simulink model "IMcontrol0"  (Simulink 10.1)
settings: Solver=ode23tb  StartTime=0.0  StopTime=10  MaxStep=1e-4  RelTol=1e-3
undefined symbols (not defined in the file or in its folder): DiscIntNeverNeededParam, Ts
libraries: powerlib x4, simulink x1
settings Model: Creator=80573  LastModifiedBy=Lenovo
settings DataIOCC: SaveFormat=Dataset
settings OptimizationCC: LifeSpan=auto
settings DebuggingCC: UnderspecifiedInitializationDetection=Simplified  MergeDetectMultiDrivingBlocksExec=error  SFUnexpectedBacktrackingDiag=error  SFNoUnconditionalDefaultTransitionDiag=error  SFExecutionAtInitializationDiag=warning
settings HardwareCC: ProdBitPerPointer=64  ProdBitPerSizeT=64  ProdBitPerPtrDiffT=64  ProdLargestAtomicFloat=Float  ProdIntDivRoundTo=Zero  ProdEndianess=LittleEndian  ProdWordSize=64  ProdHWDeviceType=Intel->x86-64 (Windows64)
settings ModelReferenceCC: PropagateSignalLabelsOutOfModel=on
settings CodeAppCC: StateflowObjectComments=off
settings GRTTargetCC: TargetLangStandard=C99 (ISO)  CombineOutputUpdateFcns=on  GRTInterface=off
settings ConfigComp: CovMetricSettings=dwe  CovHtmlReporting=off  CovSaveCumulativeToWorkspaceVar=off  CovSaveSingleToWorkspaceVar=off  CovExternalEMLEnable=on

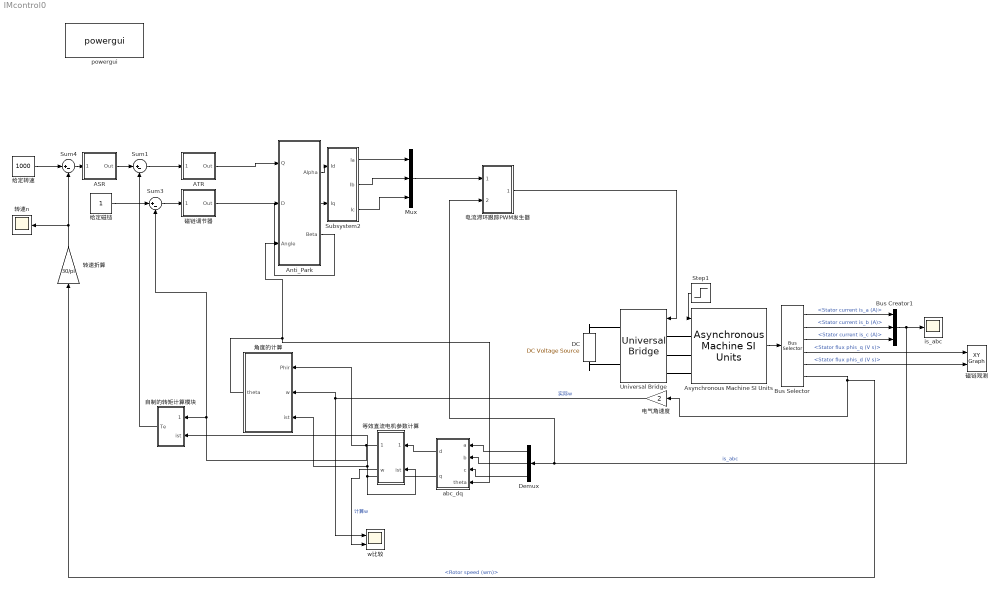
== system IMcontrol0 ==
  ASR : Subsystem  AncestorBlock=|  DialogController=POWERSYS.PowerSysDialog  mask(Discrete PI Controller){Kpw=3.8, Kiw=0.8, Ba=0, Par_Limits=[30 -30], Init=0, Ts=Ts}
      | powerlib_extras/Discrete 
      | Control Blocks/Discrete
      | PI Controller
      mask prompts: Kpw "Proportional gain (Kp):"; Kiw "Integral gain (Ki):"; Ba "feedback gain (Ba)"; Par_Limits "Output limits: [ Upper   Lower ]"; Init "Output initial value:"; Ts "Sample time:"
      mask help: This block implements a discrete PI controller.
      mask init:
      | UpperLimit=Par_Limits(1);
      | LowerLimit=Par_Limits(2);
      | power_initmask();
      mask Help: This block is part of a subset of blocks in the Extras library that does not have documentation associated with it, other than the block mask description.
      mask Display: disp('PI');
  ATR : Subsystem  AncestorBlock=|  DialogController=POWERSYS.PowerSysDialog  mask(Discrete PI Controller){Kpw=4.5, Kiw=12, Ba=0, Par_Limits=[60 -60], Init=0, Ts=Ts}
      | powerlib_extras/Discrete 
      | Control Blocks/Discrete
      | PI Controller
      mask prompts: Kpw "Proportional gain (Kp):"; Kiw "Integral gain (Ki):"; Ba "feedback gain (Ba)"; Par_Limits "Output limits: [ Upper   Lower ]"; Init "Output initial value:"; Ts "Sample time:"
      mask help: This block implements a discrete PI controller.
      mask init:
      | UpperLimit=Par_Limits(1);
      | LowerLimit=Par_Limits(2);
      | power_initmask();
      mask Help: This block is part of a subset of blocks in the Extras library that does not have documentation associated with it, other than the block mask description.
      mask Display: disp('PI');
  Anti_Park : Subsystem
  Asynchronous Machine SI Units : powerlib/Machines/Asynchronous Machine SI Units  RotorType=Squirrel-cage  PresetModel=No  MechanicalLoad=Torque Tm  ShowDetailedParameters=on  ReferenceFrame=Stationary  Units=SI  MeasurementBus=off  NominalParameters=[7500 380 50]  Stator=[0.7384 0.003045]  Rotor=[0.07402 0.003045]  Cage1=[0.4155 0.002066]  Cage2=[0.4168 0.0003495]  Lm=0.1241  Mechanical=[0.0343 0 2]  PolePairs=2  InitialConditions=[1 0 0 0 0 0 0 0]  SimulateSaturation=off  Saturation=[14.03593122, 27.81365428, 53.79336849, 72.68890987, 97.98006896, 148.6815601, 215.7428561, 302.9841135, 428.7778367 ; 230, 322, 414, 460, 506, 552, 598, 644, 690]  LoadFlowParameters=1492000  TsPowergui=0  TsBlock=-1  IterativeModel=Trapezoidal non iterative  IterativeDiscreteModel=Trapezoidal non iterative  Pmec=1.492e+006
  Bus Creator1 : BusCreator  Inputs=3
  Bus Selector : BusSelector  OutputSignals=Stator measurements.Stator current is_a (A),Stator measurements.Stator current is_b (A),Stator measurements.Stator current is_c (A),Stator measurements.Stator flux phis_q (V s),Stator measurements.Stator flux phis_d (V s),Mechanical.Rotor speed (wm)
  DC : powerlib/Electrical Sources/DC Voltage Source  Amplitude=510  Measurements=None
  Demux : Demux  Outputs=3
  Mux : Mux  Inputs=3
  Step1 : Step  After=2  SampleTime=0
  Subsystem2 : Subsystem
  Sum1 : Sum  Inputs=|+-
  Sum3 : Sum  Inputs=|+-
  Sum4 : Sum  Inputs=|+-
  Universal Bridge : powerlib/Power Electronics/Universal Bridge  Arms=3  SnubberResistance=1e5  SnubberCapacitance=inf  Device=IGBT / Diodes  Ron=1e-3  Lon=0  ForwardVoltages="[  0  0  ]"  ForwardVoltage=0  GTOparameters=[ 10e-6 , 20e-6 ]  IGBTparameters=[ 1e-6 , 2e-6 ]  Measurements=None  Measurements_2=None  converterType=Rectifier
  abc_dq : Subsystem
  is_abc : Scope
  powergui : powerlib/powergui  SimulationMode=Discrete  SampleTime=0.00001  frequency=50  Iterations=50  frequencyindice=50  Pbase=100e6  ErrMax=1e-4  UnitsV=kV  UnitsW=MW  buscounter=0  FunctionMessages=off  echomessages=off  EnableUseOfTLC=off  CurrentSourceSwitches=off  DisableSnubberDevices=off  DisableRonSwitches=off  DisableVfSwitches=off  DisplayEquations=off  AutomaticDiscreteSolvers=off  SolverType=Tustin/Backward Euler (TBE)  Interpol=off  ExternalGateDelay=off  methode=off  Ts=100  x0status=zero  SPID=on  SwTol=0  HookPort=off  NonlinearTolerance=1e-4  nMaxIteration=100  ContinueOnMaxIteration=off  RestoreLinks=warning  ResistiveCurrentMeasurement=off  Frange=[0:2:500]  Ylog=off  Xlog=on  ShowGrid=off  save=off  variable=ZData  structure=0  ZoomFFT=on  StartTime=0.0  cycles=1  DisplayStyle=1  fundamental=60  FreqAxis=off  MaxFrequency=1000  frequencyindicesteady=1  RmsSteady=1  display=off
  w比较 : Scope  NumInputPorts=2
  电气角速度 : Gain  Gain=2
  电流滞环跟踪PWM发生器 : Subsystem
  磁链观测 : simulink/Sinks/XY Graph  xmin=-1  xmax=1  ymin=-1  ymax=1  st=-1
  磁链调节器 : Subsystem  AncestorBlock=|  DialogController=POWERSYS.PowerSysDialog  mask(Discrete PI Controller){Kpw=1.8, Kiw=100, Ba=0, Par_Limits=[13 -13], Init=0, Ts=Ts}
      | powerlib_extras/Discrete 
      | Control Blocks/Discrete
      | PI Controller
      mask prompts: Kpw "Proportional gain (Kp):"; Kiw "Integral gain (Ki):"; Ba "feedback gain (Ba)"; Par_Limits "Output limits: [ Upper   Lower ]"; Init "Output initial value:"; Ts "Sample time:"
      mask help: This block implements a discrete PI controller.
      mask init:
      | UpperLimit=Par_Limits(1);
      | LowerLimit=Par_Limits(2);
      | power_initmask();
      mask Help: This block is part of a subset of blocks in the Extras library that does not have documentation associated with it, other than the block mask description.
      mask Display: disp('PI');
  等效直流电机参数计算 : Subsystem
  给定磁链 : Constant
  给定转速 : Constant  Value=1000
  自制的转矩计算模块 : Subsystem
  角度的计算 : Subsystem
  转速n : Scope
  转速折算 : Gain  Gain=30/pi
  wires:
  Step1/1 -> Asynchronous Machine SI Units/1
  abc_dq/1(d) -> 等效直流电机参数计算/1(ism)
  abc_dq/2(q) -> 自制的转矩计算模块/2(ist), 角度的计算/3(ist), 等效直流电机参数计算/2(ist)
  Sum1/1 -> ATR/1(Error)
  Sum3/1 -> 磁链调节器/1(Error)
  Sum4/1 -> ASR/1(Error)
  给定磁链/1 -> Sum3/1
  等效直流电机参数计算/1(Phir) -> 角度的计算/1(Phir), 自制的转矩计算模块/1(phir), Sum3/2
  Mux/1 -> 电流滞环跟踪PWM发生器/1(Iabc*)
  角度的计算/1(theta) -> Anti_Park/3(Angle), abc_dq/4(theta)
  Subsystem2/1(Ia) -> Mux/1
  Bus Selector/1 -> Bus Creator1/1  "<Stator current is_a (A)>"
  Bus Selector/3 -> Bus Creator1/3  "<Stator current is_c (A)>"
  Bus Selector/4 -> 磁链观测/1  "<Stator flux phis_q (V s)>"
  Bus Selector/5 -> 磁链观测/2  "<Stator flux phis_d (V s)>"
  Bus Selector/2 -> Bus Creator1/2  "<Stator current is_b (A)>"
  Bus Selector/6 -> 转速折算/1, 电气角速度/1  "<Rotor speed (wm)>"
  Bus Creator1/1 -> 电流滞环跟踪PWM发生器/2(Iabc), Demux/1, is_abc/1  "is_abc"
  Asynchronous Machine SI Units/1 -> Bus Selector/1
  电流滞环跟踪PWM发生器/1(pulse) -> Universal Bridge/1
  Demux/2 -> abc_dq/2(b)
  Demux/3 -> abc_dq/3(c)
  Demux/1 -> abc_dq/1(a)
  电气角速度/1 -> w比较/1, 角度的计算/2(w)  "实际w"
  等效直流电机参数计算/2(w) -> w比较/2  "计算w"
  磁链调节器/1(Out) -> Anti_Park/2(D)
  ATR/1(Out) -> Anti_Park/1(Q)
  Anti_Park/1(Alpha) -> Subsystem2/1(Id)
  Anti_Park/2(Beta) -> Subsystem2/2(Iq)
  给定转速/1 -> Sum4/1
  转速折算/1 -> 转速n/1, Sum4/2
  Subsystem2/3(Ic) -> Mux/3
  Subsystem2/2(Ib) -> Mux/2
  ASR/1(Out) -> Sum1/1
  自制的转矩计算模块/1(Te) -> Sum1/2
  connections:
  Universal Bridge/LConn1 -- Asynchronous Machine SI Units/LConn1
  Universal Bridge/LConn3 -- Asynchronous Machine SI Units/LConn3
  DC/LConn1 -- Universal Bridge/RConn2
  Universal Bridge/LConn2 -- Asynchronous Machine SI Units/LConn2
  DC/RConn1 -- Universal Bridge/RConn1

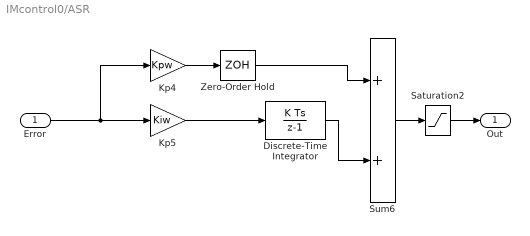
== system IMcontrol0/ASR ==
  Error : Inport  SampleTime=Ts
  Discrete-Time Integrator : DiscreteIntegrator  InitialCondition=Init  SampleTime=Ts  OutMin=[-80]  OutMax=[80]  LimitOutput=on  UpperSaturationLimit=UpperLimit  LowerSaturationLimit=LowerLimit  ICPrevOutput=DiscIntNeverNeededParam  ICPrevScaledInput=DiscIntNeverNeededParam
  Kp4 : Gain  Gain=Kpw  SaturateOnIntegerOverflow=on  SampleTime=Ts  OutDataTypeStr=Inherit: Same as input  ParamDataTypeStr=Inherit: Same as input
  Kp5 : Gain  Gain=Kiw  SaturateOnIntegerOverflow=on  SampleTime=Ts  OutDataTypeStr=Inherit: Same as input  ParamDataTypeStr=Inherit: Same as input
  Saturation2 : Saturate  UpperLimit=UpperLimit  LowerLimit=LowerLimit  SampleTime=Ts  OutMin=[-75]  OutMax=[75]
  Sum6 : Sum  InputSameDT=on  SaturateOnIntegerOverflow=on  SampleTime=Ts  OutDataTypeStr=Inherit: Same as first input
  Zero-Order Hold : ZeroOrderHold  SampleTime=Ts
  Out : Outport  SampleTime=Ts  InitialOutput=0  VectorParamsAs1DForOutWhenUnconnected=off
  wires:
  Error/1 -> Kp5/1, Kp4/1
  Zero-Order Hold/1 -> Sum6/1
  Saturation2/1 -> Out/1
  Discrete-Time Integrator/1 -> Sum6/2
  Kp4/1 -> Zero-Order Hold/1
  Kp5/1 -> Discrete-Time Integrator/1
  Sum6/1 -> Saturation2/1

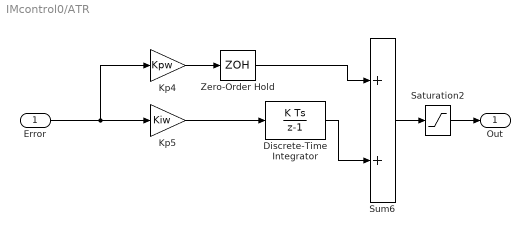
== system IMcontrol0/ATR ==
  Error : Inport  SampleTime=Ts
  Discrete-Time Integrator : DiscreteIntegrator  InitialCondition=Init  SampleTime=Ts  OutMin=[-65]  OutMax=[65]  LimitOutput=on  UpperSaturationLimit=UpperLimit  LowerSaturationLimit=LowerLimit  ICPrevOutput=DiscIntNeverNeededParam  ICPrevScaledInput=DiscIntNeverNeededParam
  Kp4 : Gain  Gain=Kpw  SaturateOnIntegerOverflow=on  SampleTime=Ts  OutDataTypeStr=Inherit: Same as input  ParamDataTypeStr=Inherit: Same as input
  Kp5 : Gain  Gain=Kiw  SaturateOnIntegerOverflow=on  SampleTime=Ts  OutDataTypeStr=Inherit: Same as input  ParamDataTypeStr=Inherit: Same as input
  Saturation2 : Saturate  UpperLimit=UpperLimit  LowerLimit=LowerLimit  SampleTime=Ts  OutMin=[-60]  OutMax=[60]
  Sum6 : Sum  InputSameDT=on  SaturateOnIntegerOverflow=on  SampleTime=Ts  OutDataTypeStr=Inherit: Same as first input
  Zero-Order Hold : ZeroOrderHold  SampleTime=Ts
  Out : Outport  SampleTime=Ts  InitialOutput=0  VectorParamsAs1DForOutWhenUnconnected=off
  wires:
  Error/1 -> Kp5/1, Kp4/1
  Zero-Order Hold/1 -> Sum6/1
  Saturation2/1 -> Out/1
  Discrete-Time Integrator/1 -> Sum6/2
  Kp4/1 -> Zero-Order Hold/1
  Kp5/1 -> Discrete-Time Integrator/1
  Sum6/1 -> Saturation2/1

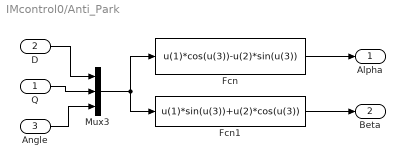
== system IMcontrol0/Anti_Park ==
  Q : Inport
  D : Inport  Port=2
  Angle : Inport  Port=3
  Fcn : Fcn  Expr=u(1)*cos(u(3))-u(2)*sin(u(3))
  Fcn1 : Fcn  Expr=u(1)*sin(u(3))+u(2)*cos(u(3))
  Mux3 : Mux  Inputs=3
  Alpha : Outport  VectorParamsAs1DForOutWhenUnconnected=off
  Beta : Outport  Port=2  VectorParamsAs1DForOutWhenUnconnected=off
  wires:
  Angle/1 -> Mux3/3
  Fcn1/1 -> Beta/1
  Mux3/1 -> Fcn1/1, Fcn/1
  Fcn/1 -> Alpha/1
  D/1 -> Mux3/1
  Q/1 -> Mux3/2

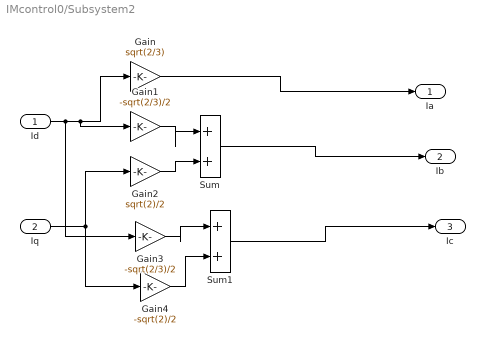
== system IMcontrol0/Subsystem2 ==
  Id : Inport
  Iq : Inport  Port=2
  Gain : Gain  Gain=sqrt(2/3)  SaturateOnIntegerOverflow=on  OutDataTypeStr=Inherit: Same as input  ParamDataTypeStr=Inherit: Same as input
  Gain1 : Gain  Gain=-sqrt(2/3)/2  SaturateOnIntegerOverflow=on  OutDataTypeStr=Inherit: Same as input  ParamDataTypeStr=Inherit: Same as input
  Gain2 : Gain  Gain=sqrt(2)/2  SaturateOnIntegerOverflow=on  OutDataTypeStr=Inherit: Same as input  ParamDataTypeStr=Inherit: Same as input
  Gain3 : Gain  Gain=-sqrt(2/3)/2  SaturateOnIntegerOverflow=on  OutDataTypeStr=Inherit: Same as input  ParamDataTypeStr=Inherit: Same as input
  Gain4 : Gain  Gain=-sqrt(2)/2  SaturateOnIntegerOverflow=on  OutDataTypeStr=Inherit: Same as input  ParamDataTypeStr=Inherit: Same as input
  Sum : Sum  Inputs=|++  SaturateOnIntegerOverflow=on
  Sum1 : Sum  Inputs=|++  SaturateOnIntegerOverflow=on
  Ia : Outport
  Ib : Outport  Port=2
  Ic : Outport  Port=3
  wires:
  Id/1 -> Gain/1, Gain1/1, Gain3/1
  Gain/1 -> Ia/1
  Iq/1 -> Gain2/1, Gain4/1
  Gain1/1 -> Sum/1
  Gain2/1 -> Sum/2
  Sum/1 -> Ib/1
  Gain3/1 -> Sum1/1
  Gain4/1 -> Sum1/2
  Sum1/1 -> Ic/1

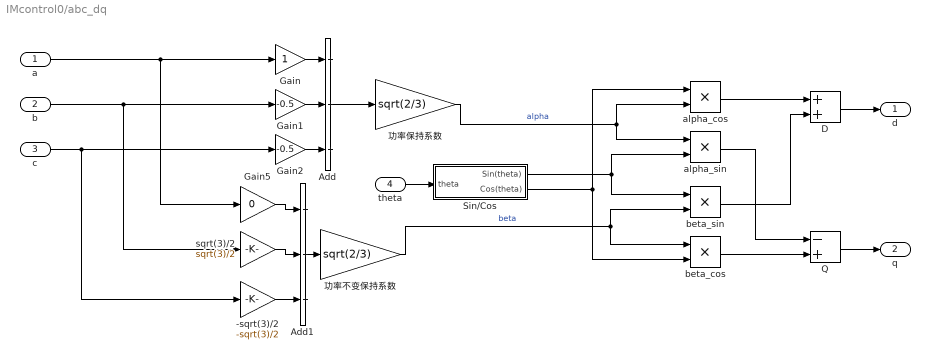
== system IMcontrol0/abc_dq ==
  a : Inport
  b : Inport  Port=2
  c : Inport  Port=3
  theta : Inport  Port=4
  -sqrt(3)/2 : Gain  Gain=-sqrt(3)/2
  Add : Sum  Inputs=3
  Add1 : Sum  Inputs=3
  D : Sum
  Gain : Gain
  Gain1 : Gain  Gain=-0.5
  Gain2 : Gain  Gain=-0.5
  Gain5 : Gain  Gain=0
  Q : Sum  Inputs=-+
  Sin/Cos : Subsystem
  alpha_cos : Product
  alpha_sin : Product
  beta_cos : Product
  beta_sin : Product
  sqrt(3)/2 : Gain  Gain=sqrt(3)/2
  功率不变保持系数 : Gain  Gain=sqrt(2/3)
  功率保持系数 : Gain  Gain=sqrt(2/3)
  d : Outport  VectorParamsAs1DForOutWhenUnconnected=off
  q : Outport  Port=2  VectorParamsAs1DForOutWhenUnconnected=off
  wires:
  功率不变保持系数/1 -> beta_cos/1, beta_sin/2  "beta"
  D/1 -> d/1
  Sin/Cos/2(Cos(theta)) -> beta_cos/2, alpha_cos/1
  alpha_sin/1 -> Q/1
  Q/1 -> q/1
  beta_sin/1 -> D/2
  beta_cos/1 -> Q/2
  Sin/Cos/1(Sin(theta)) -> beta_sin/1, alpha_sin/2
  功率保持系数/1 -> alpha_cos/2, alpha_sin/1  "alpha"
  Add1/1 -> 功率不变保持系数/1
  c/1 -> Gain2/1, -sqrt(3)/2/1
  a/1 -> Gain5/1, Gain/1
  Gain2/1 -> Add/3
  sqrt(3)/2/1 -> Add1/2
  theta/1 -> Sin/Cos/1(theta)
  b/1 -> sqrt(3)/2/1, Gain1/1
  -sqrt(3)/2/1 -> Add1/3
  Gain1/1 -> Add/2
  Gain5/1 -> Add1/1
  alpha_cos/1 -> D/1
  Add/1 -> 功率保持系数/1
  Gain/1 -> Add/1

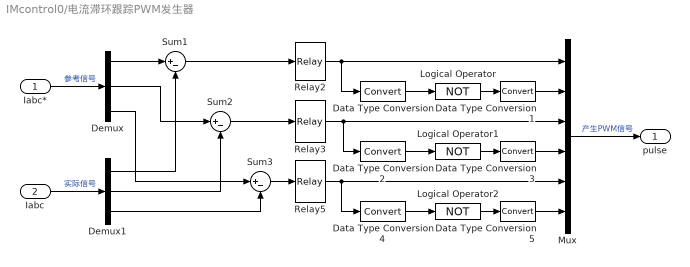
== system IMcontrol0/电流滞环跟踪PWM发生器 ==
  Iabc* : Inport
  Iabc : Inport  Port=2
  Data Type Conversion{,1..5} (6 alike) : DataTypeConversion
  Demux : Demux  Outputs=3
  Demux1 : Demux  Outputs=3
  Logical Operator : Logic  Operator=NOT  Inputs=1  AllPortsSameDT=off
  Logical Operator1 : Logic  Operator=NOT  Inputs=1  AllPortsSameDT=off
  Logical Operator2 : Logic  Operator=NOT  Inputs=1  AllPortsSameDT=off
  Mux : Mux  Inputs=6
  Relay2 : Relay  OnSwitchValue=0.2  OffSwitchValue=-0.2  ZeroCross=off
  Relay3 : Relay  OnSwitchValue=0.2  OffSwitchValue=-0.2  ZeroCross=off
  Relay5 : Relay  OnSwitchValue=0.2  OffSwitchValue=-0.2  ZeroCross=off
  Sum1 : Sum  Inputs=|+-
  Sum2 : Sum  Inputs=|+-
  Sum3 : Sum  Inputs=|+-
  pulse : Outport  VectorParamsAs1DForOutWhenUnconnected=off
  wires:
  Relay2/1 -> Data Type Conversion/1, Mux/1
  Data Type Conversion/1 -> Logical Operator/1
  Logical Operator/1 -> Data Type Conversion1/1
  Data Type Conversion1/1 -> Mux/2
  Mux/1 -> pulse/1  "产生PWM信号"
  Sum1/1 -> Relay2/1
  Demux/1 -> Sum1/1
  Demux1/3 -> Sum3/2
  Iabc/1 -> Demux1/1  "实际信号"
  Iabc*/1 -> Demux/1  "参考信号"
  Sum2/1 -> Relay3/1
  Logical Operator1/1 -> Data Type Conversion3/1
  Data Type Conversion3/1 -> Mux/4
  Data Type Conversion2/1 -> Logical Operator1/1
  Relay3/1 -> Data Type Conversion2/1, Mux/3
  Logical Operator2/1 -> Data Type Conversion5/1
  Data Type Conversion5/1 -> Mux/6
  Data Type Conversion4/1 -> Logical Operator2/1
  Relay5/1 -> Data Type Conversion4/1, Mux/5
  Sum3/1 -> Relay5/1
  Demux/2 -> Sum2/1
  Demux1/1 -> Sum1/2
  Demux1/2 -> Sum2/2
  Demux/3 -> Sum3/1

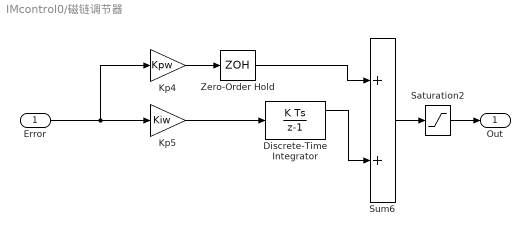
== system IMcontrol0/磁链调节器 ==
  Error : Inport  SampleTime=Ts
  Discrete-Time Integrator : DiscreteIntegrator  InitialCondition=Init  SampleTime=Ts  OutMin=[-15]  OutMax=[15]  LimitOutput=on  UpperSaturationLimit=UpperLimit  LowerSaturationLimit=LowerLimit  ShowSaturationPort=on  ShowStatePort=on  ICPrevOutput=DiscIntNeverNeededParam  ICPrevScaledInput=DiscIntNeverNeededParam
  Kp4 : Gain  Gain=Kpw  SaturateOnIntegerOverflow=on  SampleTime=Ts  OutDataTypeStr=Inherit: Same as input  ParamDataTypeStr=Inherit: Same as input
  Kp5 : Gain  Gain=Kiw  SaturateOnIntegerOverflow=on  SampleTime=Ts  OutDataTypeStr=Inherit: Same as input  ParamDataTypeStr=Inherit: Same as input
  Saturation2 : Saturate  UpperLimit=UpperLimit  LowerLimit=LowerLimit  SampleTime=Ts  OutMin=[-15]  OutMax=[15]
  Sum6 : Sum  InputSameDT=on  SaturateOnIntegerOverflow=on  SampleTime=Ts  OutDataTypeStr=Inherit: Same as first input
  Zero-Order Hold : ZeroOrderHold  SampleTime=Ts
  Out : Outport  SampleTime=Ts  InitialOutput=0  VectorParamsAs1DForOutWhenUnconnected=off
  wires:
  Error/1 -> Kp5/1, Kp4/1
  Zero-Order Hold/1 -> Sum6/1
  Saturation2/1 -> Out/1
  Discrete-Time Integrator/1 -> Sum6/2
  Kp4/1 -> Zero-Order Hold/1
  Kp5/1 -> Discrete-Time Integrator/1
  Sum6/1 -> Saturation2/1

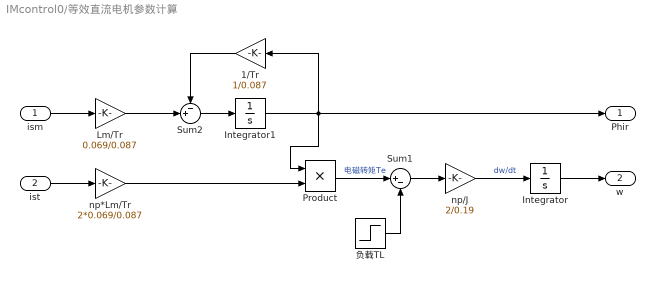
== system IMcontrol0/等效直流电机参数计算 ==
  ism : Inport
  ist : Inport  Port=2
  1/Tr : Gain  Gain=1/0.087
  Integrator : Integrator
  Integrator1 : Integrator  InitialCondition=1e-5
  Lm/Tr : Gain  Gain=0.069/0.087
  Product : Product
  Sum1 : Sum  Inputs=|+-
  Sum2 : Sum  Inputs=-+|
  np*Lm/Tr : Gain  Gain=2*0.069/0.087
  np/J : Gain  Gain=2/0.19
  负载TL : Step  Time=0.6  After=55  SampleTime=0
  Phir : Outport  VectorParamsAs1DForOutWhenUnconnected=off
  w : Outport  Port=2  VectorParamsAs1DForOutWhenUnconnected=off
  wires:
  Sum2/1 -> Integrator1/1
  Integrator1/1 -> Phir/1, Product/1, 1/Tr/1
  Sum1/1 -> np/J/1
  np*Lm/Tr/1 -> Product/2
  ism/1 -> Lm/Tr/1
  Lm/Tr/1 -> Sum2/2
  ist/1 -> np*Lm/Tr/1
  Integrator/1 -> w/1
  负载TL/1 -> Sum1/2
  np/J/1 -> Integrator/1  "dw/dt"
  Product/1 -> Sum1/1  "电磁转矩Te"
  1/Tr/1 -> Sum2/1

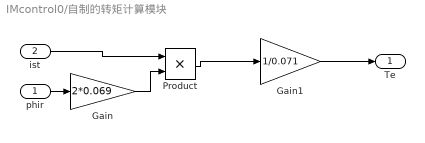
== system IMcontrol0/自制的转矩计算模块 ==
  phir : Inport
  ist : Inport  Port=2
  Gain : Gain  Gain=2*0.069
  Gain1 : Gain  Gain=1/0.071
  Product : Product
  Te : Outport  VectorParamsAs1DForOutWhenUnconnected=off
  wires:
  ist/1 -> Product/1
  Gain/1 -> Product/2
  Gain1/1 -> Te/1
  Product/1 -> Gain1/1
  phir/1 -> Gain/1

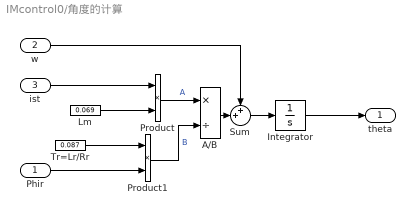
== system IMcontrol0/角度的计算 ==
  Phir : Inport
  w : Inport  Port=2
  ist : Inport  Port=3
  A/B : Product  Inputs=*/
  Integrator : Integrator
  Lm : Constant  Value=0.069
  Product : Product
  Product1 : Product
  Sum : Sum  Inputs=++|
  Tr=Lr/Rr : Constant  Value=0.087
  theta : Outport  VectorParamsAs1DForOutWhenUnconnected=off
  wires:
  ist/1 -> Product/1
  w/1 -> Sum/1
  Product/1 -> A/B/1  "A"
  Sum/1 -> Integrator/1
  Integrator/1 -> theta/1
  Product1/1 -> A/B/2  "B"
  Lm/1 -> Product/2
  A/B/1 -> Sum/2
  Phir/1 -> Product1/2
  Tr=Lr/Rr/1 -> Product1/1

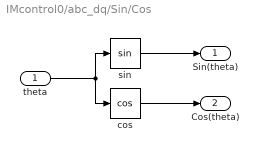
== system IMcontrol0/abc_dq/Sin/Cos ==
  theta : Inport
  cos : Trigonometry  Operator=cos
  sin : Trigonometry
  Sin(theta) : Outport  VectorParamsAs1DForOutWhenUnconnected=off
  Cos(theta) : Outport  Port=2  VectorParamsAs1DForOutWhenUnconnected=off
  wires:
  sin/1 -> Sin(theta)/1
  theta/1 -> sin/1, cos/1
  cos/1 -> Cos(theta)/1
